simulink model "vrPrueba"  (R2016b)
settings: Solver=VariableStepAuto  StartTime=0.0  StopTime=10.0  RelTol=1e-3
libraries: vrlib x2, aerospace x1
settings Model: Creator=Uxío  LastModifiedBy=Uxío

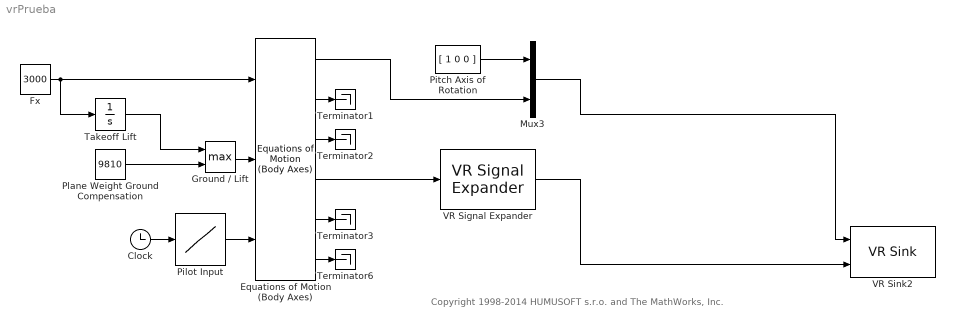
== system vrPrueba ==
  note: Copyright 1998-2014 HUMUSOFT s.r.o. and The MathWorks, Inc.
  " Equations of Motion (Body Axes)" : aerospace/3DoF Equations of Motion / Equations of Motion (Body Axes)  v_ini=0  theta_ini=0  alpha_ini=0  q_ini=0  pos_ini=[0 0]  mass=1000  Iyy=1000  g=-9.81
  Clock : Clock
  Fx : Constant  Value=3000
  Ground / Lift : MinMax  Function=max  Inputs=2  ZeroCross=off  SaturateOnIntegerOverflow=on  InputSameDT=on
  Mux3 : Mux  Inputs=2
  Pilot Input : Lookup  InputValues=[0 1 2 8 9 15]  Table=[0 0 -20 20 0 0]  SaturateOnIntegerOverflow=on
  Pitch Axis of Rotation : Constant  Value=[ 1 0 0 ]
  Plane Weight Ground Compensation : Constant  Value=9810
  Takeoff Lift : Integrator  LimitOutput=on  UpperSaturationLimit=11000  LowerSaturationLimit=-Inf  ZeroCross=off
  Terminator{1..3,6} (4 alike) : Terminator
  VR Signal Expander : vrlib/VR Signal Expander  outwidth=3  outidx=[3 2]
  VR Sink2 : vrlib/VR Sink  InstantiateOnLoad=on  SampleTime=0.1  ViewEnable=on  RemoteChange=off  RemoteView=off  FieldsWritten=Plane.rotation.4.1.1.double#Plane.translation.3.1.1.double  WorldFileName=vr01.wrl  WorldDescription=VR Plane Take-Off  AutoView=off  VideoDimensions=[]  AllowVariableSize=off  FigureProperties="{'Position', 'Name', 'Viewpoint', 'CameraBound', 'CameraDirection', 'CameraPosition', 'CameraUpVector', 'ZoomFactor', 'Antialiasing', 'Headlight', 'Lighting', 'NavPanel', 'Sound', 'StatusBar', 'Stereo3D', 'Stereo3DCameraOffset', 'Stereo3DHIT', 'ToolBar', 'Textures', 'Transparency', 'Triad', 'Wireframe', 'NavZones', 'NavMode', 'NavSpeed', 'CaptureFileFormat', 'CaptureFileName', 'Record2DCompressMethod', 'Record2DCompressQuality', 'Record2D', 'Record2DFileName', 'Record2DFPS'; [1.9210000000000000e+03   7.6000000000000000e+01   1.3660000000000000e+03   6.0100000000000000e+02], 'VR Plane Take-Off', 'Ride on the Plane', 'on', [0.0000000000000000e+00   0.0000000000000000e+00  -1.0000000000000000e+00], [0.0000000000000000e+00   0.0000000000000000e+00   0.0000000000000000e+00], [0.0000000000000000e+00   1.0000000000000000e+00   0.0000000000000000e+00], [1.0000000000000000e+00], 'on', 'on', 'on', 'halfbar', 'on', 'on', 'off', [1.0000000149011612e-01], [0.0000000000000000e+00], 'on', 'on', 'on', 'none', 'off', 'off', 'fly', 'normal', 'tif', '%f_anim_%n.tif', 'auto', [7.5000000000000000e+01], 'off', '%f_anim_%n.avi', 'auto'}"
  wires:
  Pitch Axis of Rotation/1 -> Mux3/1
  Mux3/1 -> VR Sink2/1
  VR Signal Expander/1 -> VR Sink2/2
  " Equations of Motion (Body Axes)"/2 -> Terminator1/1
  " Equations of Motion (Body Axes)"/3 -> Terminator2/1
  Ground / Lift/1 -> " Equations of Motion (Body Axes)"/2
  Takeoff Lift/1 -> Ground / Lift/1
  Plane Weight Ground Compensation/1 -> Ground / Lift/2
  Clock/1 -> Pilot Input/1
  Pilot Input/1 -> " Equations of Motion (Body Axes)"/3
  Fx/1 -> " Equations of Motion (Body Axes)"/1, Takeoff Lift/1
  " Equations of Motion (Body Axes)"/6 -> Terminator6/1
  " Equations of Motion (Body Axes)"/5 -> Terminator3/1
  " Equations of Motion (Body Axes)"/1 -> Mux3/2
  " Equations of Motion (Body Axes)"/4 -> VR Signal Expander/1
